simulink model "simulink_motor"  (R2025b)
settings: Solver=VariableStepAuto  StartTime=0.0  StopTime=10.0  RelTol=1e-3
settings Model: Creator=lhyul  LastModifiedBy=lhyul

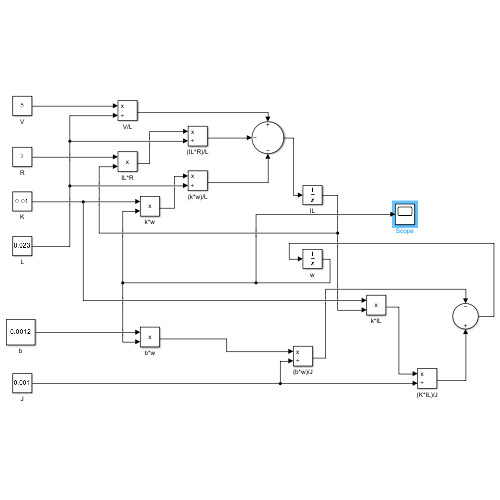
[thumbnail: Simulink's stored preview of the top-level diagram]
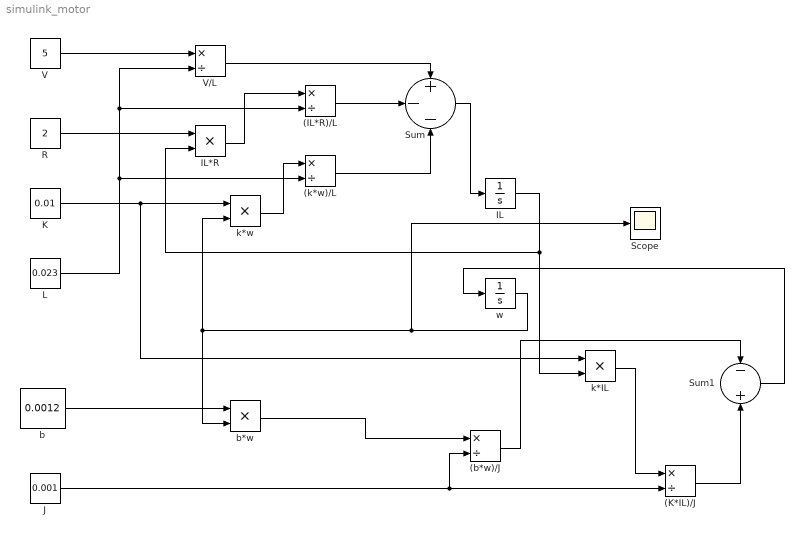
== system simulink_motor ==
  (IL*R)/L : Product  Inputs=*/
  (K*IL)/J : Product  Inputs=*/
  (b*w)/J : Product  Inputs=*/
  (k*w)/L : Product  Inputs=*/
  IL : Integrator
  IL*R : Product
  J : Constant  Value=0.001
  K : Constant  Value=0.01
  L : Constant  Value=0.023
  R : Constant  Value=2
  Scope : Scope
      settings: ActiveDisplayYMinimum=-2.5000247365856434  ActiveDisplayYMaximum=22.500222629270795
  Sum : Sum  Inputs=+--
  Sum1 : Sum  Inputs=-+
  V : Constant  Value=5
  V/L : Product  Inputs=*/
  b : Constant  Value=0.0012
  b*w : Product
  k*IL : Product
  k*w : Product
  w : Integrator
  wires:
  V/1 -> V/L/1
  L/1 -> (k*w)/L/2, (IL*R)/L/2, V/L/2
  V/L/1 -> Sum/1
  R/1 -> IL*R/1
  IL/1 -> k*IL/2, IL*R/2
  IL*R/1 -> (IL*R)/L/1
  K/1 -> k*w/1, k*IL/1
  w/1 -> Scope/1, b*w/2, k*w/2
  (IL*R)/L/1 -> Sum/2
  k*w/1 -> (k*w)/L/1
  (k*w)/L/1 -> Sum/3
  Sum1/1 -> w/1
  b/1 -> b*w/1
  b*w/1 -> (b*w)/J/1
  J/1 -> (b*w)/J/2, (K*IL)/J/2
  Sum/1 -> IL/1
  k*IL/1 -> (K*IL)/J/1
  (K*IL)/J/1 -> Sum1/2
  (b*w)/J/1 -> Sum1/1
